simulink model "problem3"  (R2020b)
settings: Solver=VariableStepAuto  StartTime=0.0  StopTime=10  MaxStep=0.00001  RelTol=1e-3
settings Model: Creator=Varun  LastModifiedBy=Varun

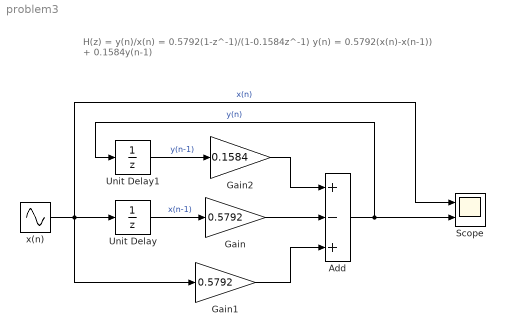
== system problem3 ==
  note: H(z) = y(n)/x(n) = 0.5792(1-z^-1)/(1-0.1584z^-1)
      | y(n) = 0.5792(x(n)-x(n-1)) + 0.1584y(n-1)
  Add : Sum  Inputs=+-+
  Gain : Gain  Gain=0.5792
  Gain1 : Gain  Gain=0.5792
  Gain2 : Gain  Gain=0.1584
  Scope : Scope  NumInputPorts=2
  Unit Delay : UnitDelay  SampleTime=-1  HasFrameUpgradeWarning=on
  Unit Delay1 : UnitDelay  SampleTime=-1  HasFrameUpgradeWarning=on
  x(n) : Sin  Frequency=8000  SampleTime=0
  wires:
  Unit Delay/1 -> Gain/1  "x(n-1)"
  Gain/1 -> Add/2
  x(n)/1 -> Scope/1, Gain1/1, Unit Delay/1  "x(n)"
  Unit Delay1/1 -> Gain2/1  "y(n-1)"
  Gain2/1 -> Add/1
  Gain1/1 -> Add/3
  Add/1 -> Scope/2, Unit Delay1/1  "y(n)"
